simulink model "top_model_24a"  (R2024a)
settings: Solver=VariableStepAuto  StartTime=0.0  StopTime=90  RelTol=1e-3  EnableMultiTasking=on
values from neighbouring files (symbols this model uses):
  target = waypoints(idx, :)'    [waypointFollower - Copy.m]    (also in waypointFollower.m)
undefined symbols (not defined in the file or in its folder): controller, gray, vehicle, X, Y, Z
libraries: sm_lib x13, nesl_utility x6, simulink x5, slpidlib x2, robotmobilelib x1
(part 2 of 2)

== matlab function top_model_24a/Motion Planning & Reference Generation (Waypoints)/MATLAB Function2 ==
  data: position_X output; position_Y output; trigger input
function [position_X, position_Y] = moveThroughCircles(trigger)
% MOVETHROUGHCIRCLES Moves through black circles with a 5-second stop.
%
% Inputs:
%   trigger: A trigger signal to advance to the next circle.
%
% Outputs:
%   position_X: The current X coordinate (column number).
%   position_Y: The current Y coordinate (row number from top).
 
persistent circleCoordinates index startTime currentState
 
% Define the coordinates of the black circles (column, row)
if isempty(circleCoordinates)
    circleCoordinates = [
        1 1; 1 2; 1 3; 1 4; 1 5; 1 6; % Column 1
        2 2; 2 3; 2 4; 2 5;           % Column 2
        3 1; 3 2; 3 3; 3 4; 3 5; 3 6; % Column 3
        4 1; 4 2; 4 3; 4 4; 4 5; 4 6; % Column 4
        5 1; 5 2; 5 3; 5 4; 5 5; 5 6; % Column 5
        6 1; 6 2; 6 3; 6 4; 6 5;       % Column 6
    ];
    index = 1;
    startTime = -inf;
    currentState = 'moving';
end
 
currentTime = get_param(bdroot, 'SimulationTime');
 
switch currentState
    case 'moving'
        % Output the current circle's coordinates
        position_X = circleCoordinates(index, 1);
        position_Y = circleCoordinates(index, 2);
 
        % Wait for a trigger to initiate the stop
        if trigger > 0
            startTime = currentTime;
            currentState = 'stopped';
        end
 
    case 'stopped'
        % Output the current circle's coordinates (still stopped)
        position_X = circleCoordinates(index, 1);
        position_Y = circleCoordinates(index, 2);
 
        % Check if the stop duration has elapsed
        if currentTime - startTime >= 5
            index = index + 1;
            if index > size(circleCoordinates, 1)
                % Optionally reset or hold the last position
                index = 1; % Loop back to the beginning
                % currentState = 'finished';
            else
                currentState = 'moving';
            end
        end
 
    case 'finished'
        % Output a final position
        position_X = circleCoordinates(end, 1);
        position_Y = circleCoordinates(end, 2);
end
